simulink library "libMdl_CarriageMisalignment"  (R2019b)
settings: Solver=VariableStepAuto  StartTime=0.0  StopTime=10.0  RelTol=1e-3
libraries: libMdl_invQuat x1, libMdl_transformVect x1
settings Model: Creator=Hanno  LastModifiedBy=Hanno

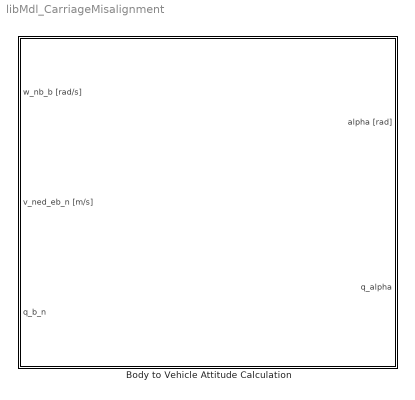
== system libMdl_CarriageMisalignment ==
  Body to Vehicle Attitude Calculation : Subsystem  mask(Waggon Bogie Misalignment Correction){mv_d_bogies=15.1}
      mask prompts: mv_d_bogies "Bogie distance:"
      mask help: see: C. Reimer, F. Müller, and E. Hinüber, "INS/GNSS/Odometer data fusion in railway applications", DGON Inertial Sensors and Systems (ISS), 2016
      mask Display:
      | str1 = sprintf('\\color{black}{\\bfBody to Vehicle Attitude Calculation}\n\n');
      | str2 = sprintf('Bogie Distance: %0.1f',mv_d_bogies);
      | 
      | str = [str1,str2];
      | 
      | text( 0.5,0.5, ...
      |       str, ...
      |       'horizontalAlignment', 'center', ...
      |       'texmode','on' ...
      |     )

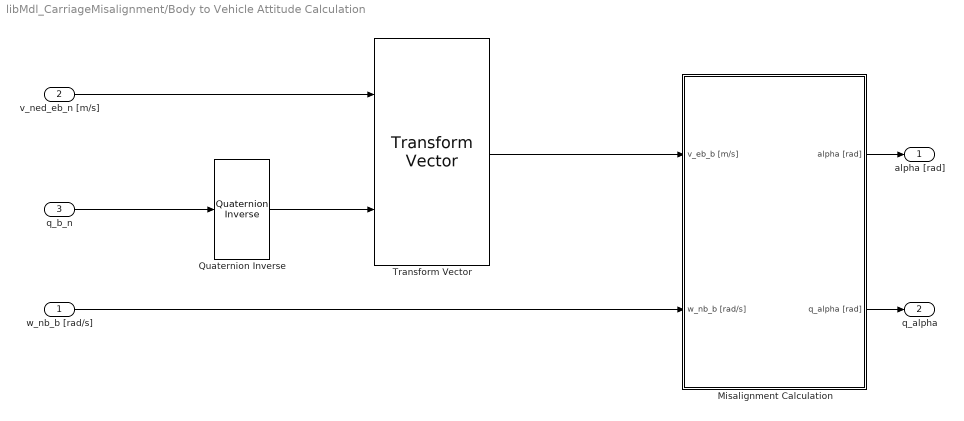
== system libMdl_CarriageMisalignment/Body to Vehicle Attitude Calculation ==
  w_nb_b [rad/s] : Inport
  v_ned_eb_n [m/s] : Inport  Port=2
  q_b_n : Inport  Port=3
  Misalignment Calculation : Subsystem
  Quaternion Inverse : libMdl_invQuat/Quaternion Inverse  SystemSampleTime=-1  Latency=0  AutoFrameSizeCalculation=off
  Transform Vector : libMdl_transformVect/Transform Vector  SystemSampleTime=-1  Latency=0  AutoFrameSizeCalculation=off
  alpha [rad] : Outport  VectorParamsAs1DForOutWhenUnconnected=off
  q_alpha : Outport  Port=2  VectorParamsAs1DForOutWhenUnconnected=off
  wires:
  Misalignment Calculation/2(q_alpha [rad]) -> q_alpha/1
  q_b_n/1 -> Quaternion Inverse/1
  Quaternion Inverse/1 -> Transform Vector/2
  v_ned_eb_n [m/s]/1 -> Transform Vector/1
  Transform Vector/1 -> Misalignment Calculation/1(v_eb_b [m/s])
  w_nb_b [rad/s]/1 -> Misalignment Calculation/2(w_nb_b [rad/s])
  Misalignment Calculation/1(alpha [rad]) -> alpha [rad]/1

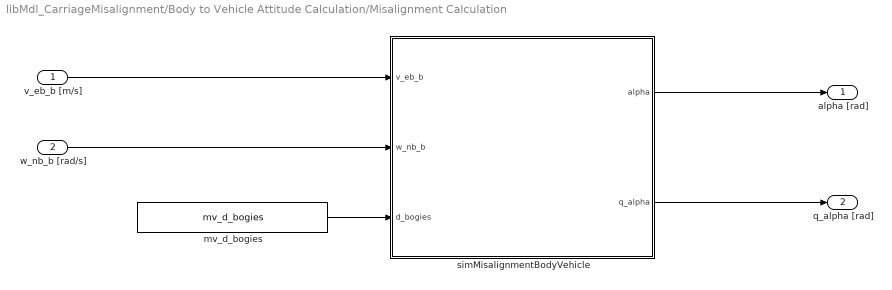
== system libMdl_CarriageMisalignment/Body to Vehicle Attitude Calculation/Misalignment Calculation ==
  v_eb_b [m/s] : Inport
  w_nb_b [rad/s] : Inport  Port=2
  mv_d_bogies : Constant  Value=mv_d_bogies
  simMisalignmentBodyVehicle : MATLAB Function  TreatAsAtomicUnit=on
  alpha [rad] : Outport  VectorParamsAs1DForOutWhenUnconnected=off
  q_alpha [rad] : Outport  Port=2  VectorParamsAs1DForOutWhenUnconnected=off
  wires:
  simMisalignmentBodyVehicle/2(q_alpha) -> q_alpha [rad]/1
  simMisalignmentBodyVehicle/1(alpha) -> alpha [rad]/1
  v_eb_b [m/s]/1 -> simMisalignmentBodyVehicle/1(v_eb_b)
  w_nb_b [rad/s]/1 -> simMisalignmentBodyVehicle/2(w_nb_b)
  mv_d_bogies/1 -> simMisalignmentBodyVehicle/3(d_bogies)

== matlab function libMdl_CarriageMisalignment/Body to Vehicle Attitude Calculation/Misalignment Calculation/simMisalignmentBodyVehicle ==
  data: v_eb_b input; alpha output; w_nb_b input; d_bogies input; q_alpha output
function [alpha,q_alpha] = simMisalignmentBodyVehicle(v_eb_b,w_nb_b,d_bogies)

% Defines _________________________________________________________________

min_turn_rate = 1e-2; % minimal detectable turn rate in rad/s
min_speed = 2 / 3.6; % minimal speed in m/s
min_radius = 60; % minimal realistic curve radius in m

% Calculations ____________________________________________________________

alpha = 0; % standard output if it is not overwritten below

v_x = v_eb_b(1);
w_z = w_nb_b(3);

if (abs(w_z) > min_turn_rate) && (abs(v_x) > min_speed)
    R = v_x/w_z;
    
    if abs(R) > min_radius
        alpha = asin( d_bogies/(2*R) );
    end % if 
end % if

q_alpha = [cos(alpha/2);0;0;sin(alpha/2)];

end % function
